simulink model "model_aio"  (Simulink 7.8)
settings: Solver=FixedStepDiscrete  SolverMode=SingleTasking  StartTime=0.0  StopTime=inf  FixedStep=0.001  RelTol=1e-3
undefined symbols (not defined in the file): another_event_name, my_event_name
libraries: opal_lib x6, rtio_opalrt_op5142ex1 x5, rtlab x3, simulink x2
settings Model: Creator=xxx  LastModifiedBy=wbernal  ExtModeTrigMode=oneshot  ExtModeArmWhenConnect=off  BufferReuse=off
settings DataIOCC: SaveOutput=off  SaveTime=off  SignalLoggingName=sigsOut
settings OptimizationCC: BlockReduction=off  BooleanDataType=off  InlineInvariantSignals=on  OptimizeBlockIOStorage=off  BufferReuse=off  ExpressionFolding=off  LocalBlockOutputs=off  InitFltsAndDblsToZero=on
settings DebuggingCC: AlgebraicLoopMsg=error  SaveWithParameterizedLinksMsg=none  SignalResolutionControl=TryResolveAllWithWarning  SolverPrmCheckMsg=none  MultiTaskDSMMsg=warning  MultiTaskCondExecSysMsg=none  FcnCallInpInsideContextMsg=Use local settings  StrictBusMsg=None
settings HardwareCC: TargetIntDivRoundTo=Zero  TargetEndianess=LittleEndian  TargetHWDeviceType=MATLAB Host  ProdEqTarget=off
settings RTWCC: IncludeERTFirstTime=on
settings GRTTargetCC: TargetFcnLib=ansi_tfl_tmw.mat

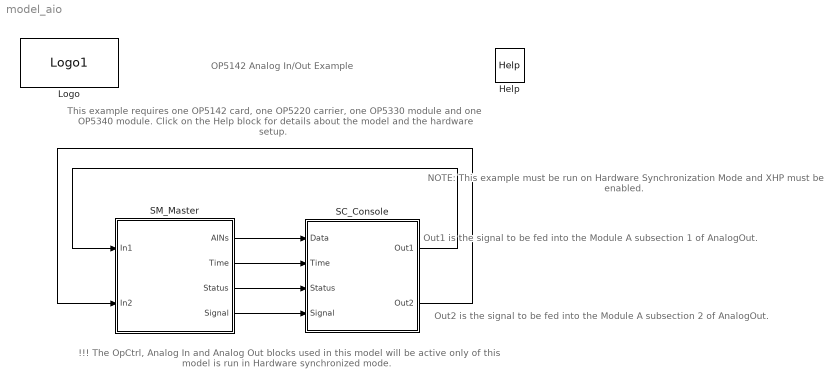
== system model_aio ==
  note: OP5142 Analog In/Out Example
  note: This example requires one OP5142 card, one OP5220 carrier, one OP5330 module and one OP5340 module.
      | Click on the Help block for details about the model and the hardware setup.
  note: !!! The OpCtrl, Analog In and Analog Out blocks used in this model will be active
      | only of this model is run in Hardware synchronized mode.
  note: NOTE: This example must be run on Hardware
      | Synchronization Mode and XHP must be enabled.
  note: Out1 is the signal to be fed into the
      | Module A subsection 1 of AnalogOut.
  note: Out2 is the signal to be fed into the
      | Module A subsection 2 of AnalogOut.
  Help : opal_lib/Help  docfile=../help/help.html
  Logo : opal_lib/Logo1  vide=[]
  SC_Console : Subsystem
  SM_Master : Subsystem
  wires:
  SM_Master/1(AINs) -> SC_Console/1(Data)
  SM_Master/2(Time) -> SC_Console/2(Time)
  SM_Master/3(Status) -> SC_Console/3(Status)
  SC_Console/1(Out1) -> SM_Master/1(In1)
  SM_Master/4(Signal) -> SC_Console/4(Signal)
  SC_Console/2(Out2) -> SM_Master/2(In2)

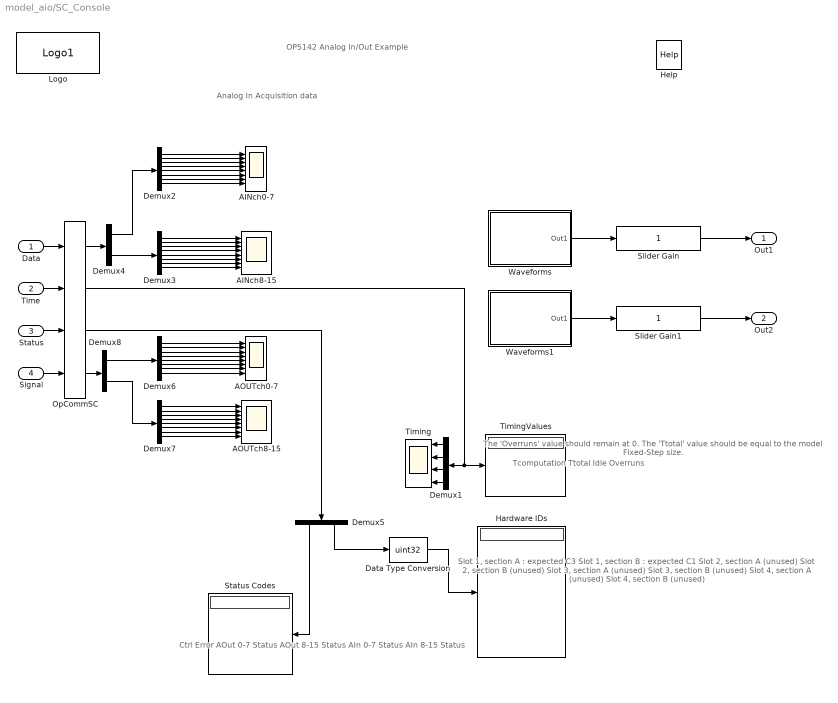
== system model_aio/SC_Console ==
  note: Tcomputation
      | Ttotal
      | Idle
      | Overruns
  note: The 'Overruns' value should remain at 0.
      | The 'Ttotal' value should be equal to the
      | model Fixed-Step size.
  note: OP5142 Analog In/Out Example
  note: Ctrl Error
      | AOut 0-7 Status
      | AOut 8-15 Status
      | AIn 0-7 Status
      | AIn 8-15 Status
  note: Slot 1, section A : expected C3
      | Slot 1, section B : expected C1
      | Slot 2, section A (unused)
      | Slot 2, section B (unused)
      | Slot 3, section A (unused)
      | Slot 3, section B (unused)
      | Slot 4, section A (unused)
      | Slot 4, section B (unused)
  note: Analog In Acquisition data
  Data : Inport
  Time : Inport  Port=2
  Status : Inport  Port=3
  Signal : Inport  Port=4
  AINch0-7 : Scope  NumInputPorts=8
      settings: TimeRange=20  YMin=-1.5~-5~-5~-5~-5~-5~-5~-5  YMax=3~5~5~5~5~5~5~5
  AINch8-15 : Scope  NumInputPorts=8
      settings: TimeRange=20  YMin=-1.5~-5~-5~-5~-5~-5~-5~-5  YMax=3~5~5~5~5~5~5~5  SaveName=ScopeData2
  AOUTch0-7 : Scope  NumInputPorts=8
      settings: TimeRange=20  YMin=-1.5~-5~-5~-5~-5~-5~-5~-5  YMax=3~5~5~5~5~5~5~5  SaveName=ScopeData3
  AOUTch8-15 : Scope  NumInputPorts=8
      settings: TimeRange=20  YMin=-1.5~-5~-5~-5~-5~-5~-5~-5  YMax=3~5~5~5~5~5~5~5  SaveName=ScopeData4
  Data Type Conversion : DataTypeConversion  OutDataTypeStr=uint32
  Demux1 : Demux
  Demux{2..3,6..7} (4 alike) : Demux  Outputs=8
  Demux4 : Demux  Outputs=2
  Demux5 : Demux  Outputs=[5 8]
  Demux8 : Demux  Outputs=2
  Hardware IDs : Display
      settings: Format=hex (Stored Integer)  Decimation=100
  Help : opal_lib/Help  docfile=../help/help.html
  Logo : opal_lib/Logo1  vide=[]
  OpCommSC : rtlab/OpComm  nbport=4  groupe_acq=1  subsys_rate=0  st=0  Synchronization=off  Interpolation=off  Threshold=1.0  Missed_Data=off  Sim_Time=off  Samples=off  dynSigOut=off  from_console=0  warning_done=off  writeOpCommFile=off  Offset=off
  Slider Gain : simulink/Math Operations/Slider Gain  low=0  gain=1  high=2
  Slider Gain1 : simulink/Math Operations/Slider Gain  low=0  gain=1  high=2
  Status Codes : Display
      settings: Decimation=100
  Timing : Scope  NumInputPorts=4
      settings: TimeRange=10  YMin=-300~-25~-5~-5  YMax=300~25~5~5  MaxDataPoints=20000
  TimingValues : Display
      settings: Decimation=100
  Waveforms : Subsystem
  Waveforms1 : Subsystem
  Out1 : Outport
  Out2 : Outport  Port=2
  wires:
  Data/1 -> OpCommSC/1
  Demux1/1 -> Timing/1
  Demux1/2 -> Timing/2
  Demux1/3 -> Timing/3
  Demux1/4 -> Timing/4
  Time/1 -> OpCommSC/2
  OpCommSC/1 -> Demux4/1
  OpCommSC/2 -> TimingValues/1, Demux1/1
  Status/1 -> OpCommSC/3
  OpCommSC/3 -> Demux5/1
  Demux5/1 -> Status Codes/1
  Demux5/2 -> Data Type Conversion/1
  Data Type Conversion/1 -> Hardware IDs/1
  Signal/1 -> OpCommSC/4
  OpCommSC/4 -> Demux8/1
  Waveforms/1(Out1) -> Slider Gain/1
  Slider Gain/1 -> Out1/1
  Demux4/1 -> Demux2/1
  Demux2/1 -> AINch0-7/1
  Demux2/2 -> AINch0-7/2
  Demux2/3 -> AINch0-7/3
  Demux2/4 -> AINch0-7/4
  Demux3/1 -> AINch8-15/1
  Demux3/2 -> AINch8-15/2
  Demux3/3 -> AINch8-15/3
  Demux3/4 -> AINch8-15/4
  Demux4/2 -> Demux3/1
  Demux2/5 -> AINch0-7/5
  Demux2/6 -> AINch0-7/6
  Demux2/7 -> AINch0-7/7
  Demux2/8 -> AINch0-7/8
  Demux3/5 -> AINch8-15/5
  Demux3/6 -> AINch8-15/6
  Demux3/7 -> AINch8-15/7
  Demux3/8 -> AINch8-15/8
  Demux8/1 -> Demux6/1
  Demux7/1 -> AOUTch8-15/1
  Demux7/2 -> AOUTch8-15/2
  Demux7/3 -> AOUTch8-15/3
  Demux7/4 -> AOUTch8-15/4
  Demux8/2 -> Demux7/1
  Demux7/5 -> AOUTch8-15/5
  Demux7/6 -> AOUTch8-15/6
  Demux7/7 -> AOUTch8-15/7
  Demux7/8 -> AOUTch8-15/8
  Demux6/1 -> AOUTch0-7/1
  Demux6/2 -> AOUTch0-7/2
  Demux6/3 -> AOUTch0-7/3
  Demux6/4 -> AOUTch0-7/4
  Demux6/5 -> AOUTch0-7/5
  Demux6/6 -> AOUTch0-7/6
  Demux6/7 -> AOUTch0-7/7
  Demux6/8 -> AOUTch0-7/8
  Waveforms1/1(Out1) -> Slider Gain1/1
  Slider Gain1/1 -> Out2/1

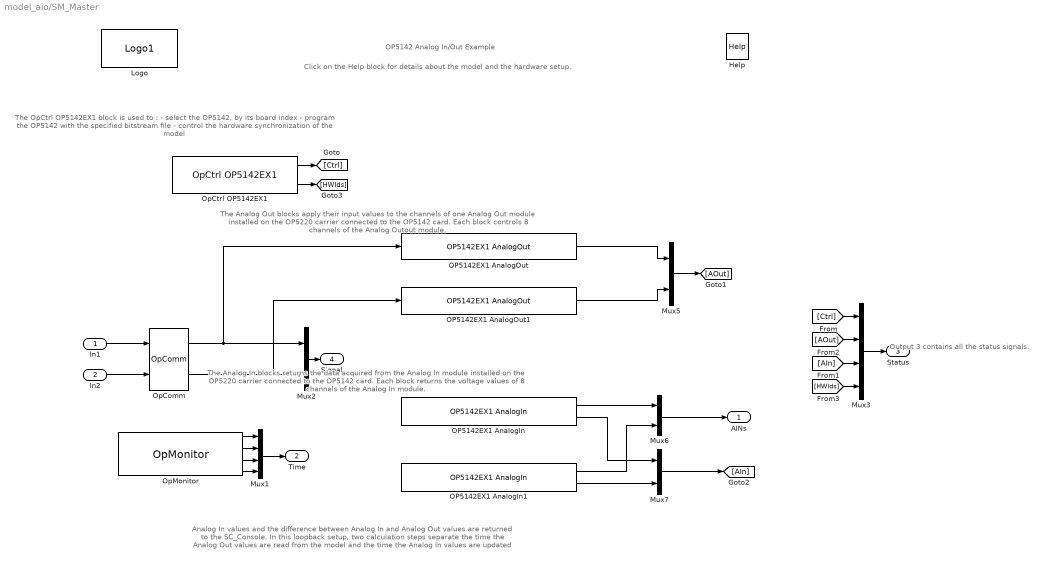
== system model_aio/SM_Master ==
  note: Click on the Help block for details about the model and the hardware setup.
  note: The OpCtrl OP5142EX1 block is used to :
      | - select the OP5142, by its board index
      | - program the OP5142 with the specified bitstream file
      | - control the hardware synchronization of the model
  note: OP5142 Analog In/Out Example
  note: The Analog Out blocks apply their input values to the channels of one Analog Out module installed on
      | the OP5220 carrier connected to the OP5142 card.
      | Each block controls 8 channels of the Analog Outout module.
  note: Analog In values and the difference between Analog In and Analog Out values are returned to the SC_Console.
      | In this loopback setup, two calculation steps separate the time the Analog Out values are read from the model and the time the
      | Analog In values are updated
  note: The Analog In blocks returns the data acquired from the Analog In module installed on the OP5220 carrier
      | connected to the OP5142 card.
      | Each block returns the voltage values of 8 channels of the Analog In module.
  note: Output 3 contains all
      | the status signals.
  In1 : Inport
  In2 : Inport  Port=2
  Help : opal_lib/Help  docfile=../help/help.html
  Logo : opal_lib/Logo1  vide=[]
  Mux1 : Mux
  Mux{2,5..7} (4 alike) : Mux  Inputs=2
  Mux3 : Mux  Inputs=[1 2 2 8]
  OP5142EX1 AnalogIn : rtio_opalrt_op5142ex1/OP5142EX1 AnalogIn  CtrlName='OP5142EX1 Ctrl'  portNb=5  FcnNos=Slot 1 Module B Subsection 1  size=16  maxcount=8  count=8  numchan=8  sampleTime=0
      settings: AttributesFormatString=%<CtrlName>
  OP5142EX1 AnalogIn1 : rtio_opalrt_op5142ex1/OP5142EX1 AnalogIn  CtrlName='OP5142EX1 Ctrl'  portNb=6  FcnNos=Slot 1 Module B Subsection 2  size=16  maxcount=8  count=8  numchan=8  sampleTime=0
      settings: AttributesFormatString=%<CtrlName>
  OP5142EX1 AnalogOut : rtio_opalrt_op5142ex1/OP5142EX1 AnalogOut  CtrlName='OP5142EX1 Ctrl'  portNb=1  FcnNos=Slot 1 Module A Subsection 1  size=16  maxcount=8  count=8  numchan=8  israngeinput=off  voltagerange=[-16 ... 16]  slot=0  side=0  mismatch=0  slotside=Slot_1_Module_A
      settings: AttributesFormatString=%<CtrlName>
  OP5142EX1 AnalogOut1 : rtio_opalrt_op5142ex1/OP5142EX1 AnalogOut  CtrlName='OP5142EX1 Ctrl'  portNb=2  FcnNos=Slot 1 Module A Subsection 2  size=16  maxcount=8  count=8  numchan=8  israngeinput=off  voltagerange=[-16 ... 16]  slot=0  side=0  mismatch=0  slotside=Slot_1_Module_A
      settings: AttributesFormatString=%<CtrlName>
  OpComm : rtlab/OpComm  nbport=2  groupe_acq=1  subsys_rate=0  st=0  Synchronization=on  Interpolation=on  Threshold=1.0  Missed_Data=off  Sim_Time=off  Samples=off  dynSigOut=off  from_console=1  warning_done=off  writeOpCommFile=off  Offset=off
  OpCtrl OP5142EX1 : rtio_opalrt_op5142ex1/OpCtrl OP5142EX1  CtrlName='OP5142EX1 Ctrl'  boardid=0  BitstreamFilename=OP5142_1-EX-0000-2_1_3_57-OP5142_8DIO_8TSDIO_6QEIO_16AIO-01-01.bin  numconfig=-1  mode=Master  externalClock=off  decimRtsi=0  calibIO=off  SampleTime=0  loadinport=-1
  OpMonitor : rtlab/Monitoring/OpMonitor  compute_time=on  real_step=on  idle_time=on  nb_overruns=on  user_time=off  user_name=my_event_name,another_event_name
  AINs : Outport
  Time : Outport  Port=2
  Status : Outport  Port=3
  Signal : Outport  Port=4
  wires:
  OpMonitor/1 -> Mux1/1
  OpMonitor/2 -> Mux1/2
  OpMonitor/3 -> Mux1/3
  OpMonitor/4 -> Mux1/4
  Mux1/1 -> Time/1
  OpCtrl OP5142EX1/1 -> [Ctrl]
  OpCtrl OP5142EX1/2 -> [HWIds]
  [Ctrl] -> Mux3/1
  [AOut] -> Mux3/2
  [AIn] -> Mux3/3
  Mux3/1 -> Status/1
  OP5142EX1 AnalogIn/2 -> Mux7/1
  OP5142EX1 AnalogOut/1 -> Mux5/1
  OP5142EX1 AnalogOut1/1 -> Mux5/2
  Mux5/1 -> [AOut]
  Mux6/1 -> AINs/1
  OP5142EX1 AnalogIn/1 -> Mux6/1
  OP5142EX1 AnalogIn1/1 -> Mux6/2
  Mux7/1 -> [AIn]
  OP5142EX1 AnalogIn1/2 -> Mux7/2
  [HWIds] -> Mux3/4
  OpComm/1 -> OP5142EX1 AnalogOut/1, Mux2/1
  In1/1 -> OpComm/1
  In2/1 -> OpComm/2
  OpComm/2 -> OP5142EX1 AnalogOut1/1, Mux2/2
  Mux2/1 -> Signal/1

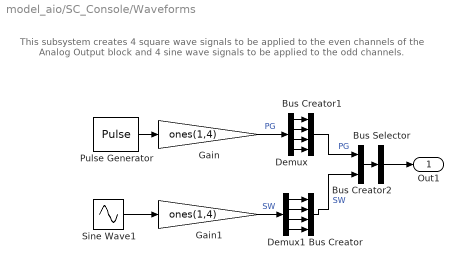
== system model_aio/SC_Console/Waveforms ==
  note: This subsystem creates 4 square wave signals to be applied to
      | the even channels of the Analog Output block and 4 sine wave
      | signals to be applied to the odd channels.
  Bus Creator : BusCreator
  Bus Creator1 : BusCreator
  Bus Creator2 : BusCreator  Inputs=2
  Bus Selector : BusSelector  OutputSignals=PG.signal1,SW.signal1,PG.signal2,SW.signal2,PG.signal3,SW.signal3,PG.signal4,SW.signal4  OutputAsBus=on
  Demux : Demux
  Demux1 : Demux
  Gain : Gain  Gain=ones(1,4)  SaturateOnIntegerOverflow=on  OutDataTypeStr=Inherit: Same as input  ParamDataTypeStr=Inherit: Same as input
  Gain1 : Gain  Gain=ones(1,4)  SaturateOnIntegerOverflow=on  OutDataTypeStr=Inherit: Same as input  ParamDataTypeStr=Inherit: Same as input
  Pulse Generator : DiscretePulseGenerator  PulseType=Time based  Period=1  PulseWidth=50
  Sine Wave1 : Sin  Frequency=10
  Out1 : Outport
  wires:
  Sine Wave1/1 -> Gain1/1
  Pulse Generator/1 -> Gain/1
  Gain/1 -> Demux/1  "PG"
  Bus Creator2/1 -> Bus Selector/1
  Bus Creator1/1 -> Bus Creator2/1  "PG"
  Bus Creator/1 -> Bus Creator2/2  "SW"
  Bus Selector/1 -> Out1/1
  Demux/1 -> Bus Creator1/1
  Demux/2 -> Bus Creator1/2
  Demux/3 -> Bus Creator1/3
  Demux/4 -> Bus Creator1/4
  Gain1/1 -> Demux1/1  "SW"
  Demux1/1 -> Bus Creator/1
  Demux1/2 -> Bus Creator/2
  Demux1/3 -> Bus Creator/3
  Demux1/4 -> Bus Creator/4

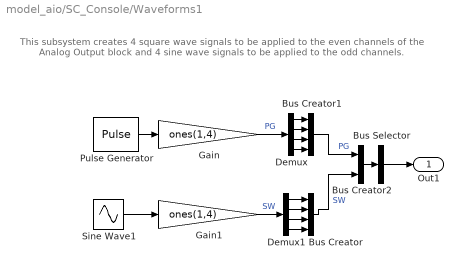
== system model_aio/SC_Console/Waveforms1 ==
  note: This subsystem creates 4 square wave signals to be applied to
      | the even channels of the Analog Output block and 4 sine wave
      | signals to be applied to the odd channels.
  Bus Creator : BusCreator
  Bus Creator1 : BusCreator
  Bus Creator2 : BusCreator  Inputs=2
  Bus Selector : BusSelector  OutputSignals=PG.signal1,SW.signal1,PG.signal2,SW.signal2,PG.signal3,SW.signal3,PG.signal4,SW.signal4  OutputAsBus=on
  Demux : Demux
  Demux1 : Demux
  Gain : Gain  Gain=ones(1,4)  SaturateOnIntegerOverflow=on  OutDataTypeStr=Inherit: Same as input  ParamDataTypeStr=Inherit: Same as input
  Gain1 : Gain  Gain=ones(1,4)  SaturateOnIntegerOverflow=on  OutDataTypeStr=Inherit: Same as input  ParamDataTypeStr=Inherit: Same as input
  Pulse Generator : DiscretePulseGenerator  PulseType=Time based  Period=1  PulseWidth=50
  Sine Wave1 : Sin  Frequency=10
  Out1 : Outport
  wires:
  Sine Wave1/1 -> Gain1/1
  Pulse Generator/1 -> Gain/1
  Gain/1 -> Demux/1  "PG"
  Bus Creator2/1 -> Bus Selector/1
  Bus Creator1/1 -> Bus Creator2/1  "PG"
  Bus Creator/1 -> Bus Creator2/2  "SW"
  Bus Selector/1 -> Out1/1
  Demux/1 -> Bus Creator1/1
  Demux/2 -> Bus Creator1/2
  Demux/3 -> Bus Creator1/3
  Demux/4 -> Bus Creator1/4
  Gain1/1 -> Demux1/1  "SW"
  Demux1/1 -> Bus Creator/1
  Demux1/2 -> Bus Creator/2
  Demux1/3 -> Bus Creator/3
  Demux1/4 -> Bus Creator/4
